simulink model "satelliteModel"  (R2018a)
settings: Solver=VariableStepAuto  StartTime=0.0  StopTime=10.0  RelTol=1e-3
values from neighbouring files (symbols this model uses):
  Ap = [0 1 0 0; 0 0 1 0; 0 0 0 1; -a4 -a3 -a2 -a1]    [SatelliteControl.m]
  Bp = [0; 0; 0; b ]    [SatelliteControl.m]
  K1 = acker(Ap,Bp,p)    [SatelliteControl.m]
settings Model: Creator=007  LastModifiedBy=007

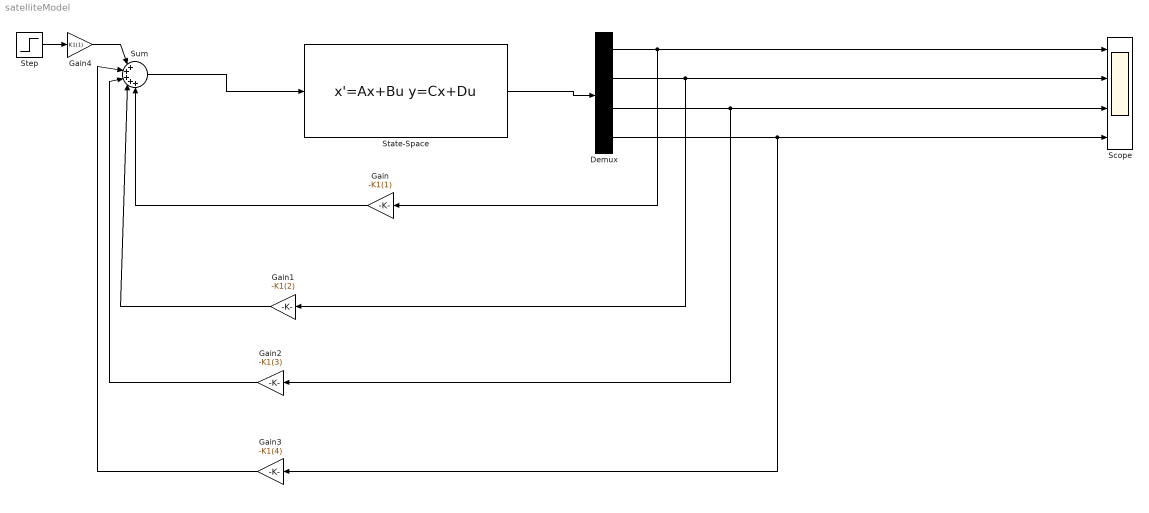
== system satelliteModel ==
  Demux : Demux
  Gain : Gain  Gain=-K1(1)
  Gain1 : Gain  Gain=-K1(2)
  Gain2 : Gain  Gain=-K1(3)
  Gain3 : Gain  Gain=-K1(4)
  Gain4 : Gain  Gain=K1(1)
  Scope : Scope  NumInputPorts=4
  State-Space : StateSpace  A=Ap  B=Bp  C=[1 0 0 0; 0 1 0 0; 0 0 1 0; 0 0 0 1]  D=[0; 0 ; 0 ; 0]  InitialCondition=0
  Step : Step  Time=0  SampleTime=0
  Sum : Sum  Inputs=|+++++
  wires:
  Gain3/1 -> Sum/2
  Demux/1 -> Gain/1, Scope/1
  Sum/1 -> State-Space/1
  Step/1 -> Gain4/1
  State-Space/1 -> Demux/1
  Demux/2 -> Gain1/1, Scope/2
  Demux/4 -> Gain3/1, Scope/4
  Demux/3 -> Gain2/1, Scope/3
  Gain/1 -> Sum/5
  Gain2/1 -> Sum/3
  Gain1/1 -> Sum/4
  Gain4/1 -> Sum/1
